simulink model "Projekt_FARE2_SS19_template_2015a"  (R2015a)
settings: Solver=ode4  SolverMode=SingleTasking  StartTime=0  StopTime=5  FixedStep=0.001  MaxStep=0.001  MinStep=1e-6  RelTol=1e-3  AbsTol=1e-3
PostLoadFcn:
  | %plot(Pos_x(:,2),Pos_y(:,2));
  | %xlabel('x(m)');
  | %ylabel('y(m)');
StopFcn:
  | %plot(Pos_x(:,2),Pos_y(:,2));
  | %xlabel('x(m)');
  | %ylabel('y(m)');
values from neighbouring files (symbols this model uses):
  delta_condi = 2    [init.m]
  K = place(A,B1,P)    [init.m]
  K10 = place(A10,B1,P)    [init.m]
  k3_condi = 1    [init.m]
  steig = 0.03    [init.m]
  v_condi = 0    [init.m]
  vorsteur_condi = 0    [init.m]
undefined symbols (not defined in the file or in its folder): in, sigbuilder_block
libraries: simulink x1
settings Model: Creator=vivgove  LastModifiedBy=eason
settings SolverCC: InitialStep=0.001  MaxOrder=3  AutoInsertRateTranBlk=on  InsertRTBMode=Never (minimum delay)
settings DataIOCC: LimitDataPoints=off  SignalLoggingSaveFormat=ModelDataLogs  SaveOutput=off  SignalLogging=off  SaveTime=off  OutputOption=SpecifiedOutputTimes  OutputTimes=[time]
settings OptimizationCC: InlineParams=on  ExpressionDepthLimit=2147483647  EfficientMapNaN2IntZero=off
settings DebuggingCC: UnderspecifiedInitializationDetection=Classic  MergeDetectMultiDrivingBlocksExec=none  SolverPrmCheckMsg=warning  FcnCallInpInsideContextMsg=EnableAllAsWarning  StateNameClashWarn=warning
settings HardwareCC: TargetBitPerLong=64  TargetBitPerPointer=64  TargetLongLongMode=on  TargetIntDivRoundTo=Zero  TargetEndianess=LittleEndian  TargetWordSize=64  TargetHWDeviceType=MATLAB Host  ProdEqTarget=off
settings CodeAppCC: MaxIdLength=128
settings GRTTargetCC: GeneratePreprocessorConditionals=Use local settings  CombineOutputUpdateFcns=off  GRTInterface=on

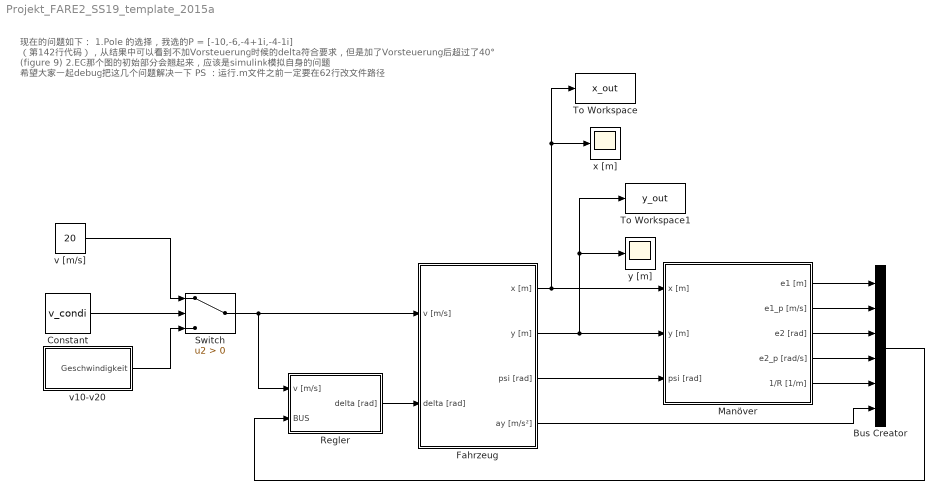
== system Projekt_FARE2_SS19_template_2015a ==
  note: 现在的问题如下：
      | 1.Pole 的选择，我选的P = [-10,-6,-4+1i,-4-1i] （第142行代码），从结果中可以看到不加Vorsteuerung时候的delta符合要求，但是加了Vorsteuerung后超过了40° (figure 9)
      | 2.EG那个图的初始部分会翘起来，应该是simulink模拟自身的问题
      |
      | 希望大家一起debug把这几个问题解决一下
      |
      | PS ：运行.m文件之前一定要在62行改文件路径
  Bus Creator : BusCreator  Inputs=6
  Constant : Constant  Value=v_condi
  Fahrzeug : Subsystem
  Manöver : Subsystem
  Regler : Subsystem
  Switch : Switch  Criteria=u2 > Threshold
  To Workspace : ToWorkspace  VariableName=x_out  SampleTime=-1
  To Workspace1 : ToWorkspace  VariableName=y_out  SampleTime=-1
  v [m/s] : Constant  Value=20
  v10-v20 : Subsystem  Tag=STV Subsys  LoadFcn=sigbuilder_block('load');  StartFcn=sigbuilder_block('start');  StopFcn=sigbuilder_block('stop');  ClipboardFcn=sigbuilder_block('clipboard');  mask(Sigbuilder block){}
      mask help: Simulink:masks:SigbuilderBlock_MD
      mask init:
      | if ~strcmp(get_param(bdroot(gcbh),'SimulationStatus'),'stopped') tuvar = sigbuilder_block('maskInit'); end
      settings: CopyFcn=sigbuilder_block('copy');  DeleteFcn=sigbuilder_block('delete');  ModelCloseFcn=sigbuilder_block('modelClose');  PreSaveFcn=sigbuilder_block('preSave');  PauseFcn=sigbuilder_block('pause');  ContinueFcn=sigbuilder_block('continue');  NameChangeFcn=sigbuilder_block('namechange');  OpenFcn=sigbuilder_block('open',[437.6 199.2 550.4 400 ]);  CloseFcn=sigbuilder_block('close');
      mask Display: plot(0, 0, 100, 100,[2, 2, 32, 32, 2], [68, 8, 8, 68, 68],[32, 2], [38, 38], [32, 19, 2],[53, 60, 44], [32, 17, 17, 2],[16, 16, 31, 31]);txt = getActiveGroup(gcbh);text(2, 100, txt,'verticalAlignment', 'top');
  x [m] : Scope
      settings: TimeRange=auto  MaxDataPoints=5000  SaveName=Pos_x  YMin=-9.34293  YMax=84.08636  SampleTime=-1  DataFormat=Array
  y [m] : Scope
      settings: TimeRange=auto  MaxDataPoints=5000  SaveName=Pos_y  YMin=-1.28728  YMax=1.75939  SampleTime=-1  DataFormat=Array
  wires:
  Manöver/1(e1 [m]) -> Bus Creator/1
  Manöver/2(e1_p [m/s]) -> Bus Creator/2
  Manöver/3(e2 [rad]) -> Bus Creator/3
  Manöver/4(e2_p [rad/s]) -> Bus Creator/4
  Manöver/5(1/R [1/m]) -> Bus Creator/5
  Bus Creator/1 -> Regler/2(BUS)
  Fahrzeug/1(x [m]) -> Manöver/1(x [m]), To Workspace/1, x [m]/1
  Fahrzeug/2(y [m]) -> Manöver/2(y [m]), y [m]/1, To Workspace1/1
  Regler/1(delta [rad]) -> Fahrzeug/2(delta [rad])
  Fahrzeug/3(psi [rad]) -> Manöver/3(psi [rad])
  Fahrzeug/4(ay [m/s²]) -> Bus Creator/6
  Switch/1 -> Fahrzeug/1(v [m/s]), Regler/1(v [m/s])
  Constant/1 -> Switch/2
  v [m/s]/1 -> Switch/1
  v10-v20/1(Geschwindigkeit) -> Switch/3

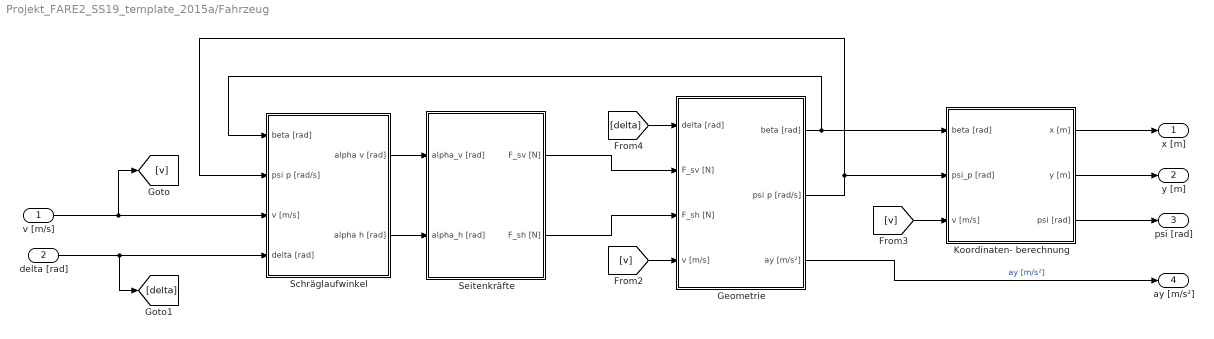
== system Projekt_FARE2_SS19_template_2015a/Fahrzeug ==
  v [m/s] : Inport
  delta [rad] : Inport  Port=2
  Geometrie : Subsystem
  Koordinaten- berechnung : Subsystem
  Schräglaufwinkel : Subsystem
  Seitenkräfte : Subsystem
  x [m] : Outport
  y [m] : Outport  Port=2
  psi [rad] : Outport  Port=3
  ay [m/s²] : Outport  Port=4
  wires:
  [v] -> Koordinaten- berechnung/3(v [m/s])
  delta [rad]/1 -> Schräglaufwinkel/4(delta [rad]), [delta]
  [v] -> Geometrie/4(v [m/s])
  [delta] -> Geometrie/1(delta [rad])
  v [m/s]/1 -> Schräglaufwinkel/3(v [m/s]), [v]
  Seitenkräfte/2(F_sh [N]) -> Geometrie/3(F_sh [N])
  Koordinaten- berechnung/3(psi [rad]) -> psi [rad]/1
  Koordinaten- berechnung/1(x [m]) -> x [m]/1
  Geometrie/2(psi p [rad/s]) -> Schräglaufwinkel/2(psi p [rad/s]), Koordinaten- berechnung/2(psi_p [rad])
  Schräglaufwinkel/2(alpha h [rad]) -> Seitenkräfte/2(alpha_h [rad])
  Koordinaten- berechnung/2(y [m]) -> y [m]/1
  Seitenkräfte/1(F_sv [N]) -> Geometrie/2(F_sv [N])
  Geometrie/1(beta [rad]) -> Koordinaten- berechnung/1(beta [rad]), Schräglaufwinkel/1(beta [rad])
  Schräglaufwinkel/1(alpha v [rad]) -> Seitenkräfte/1(alpha_v [rad])
  Geometrie/3(ay [m/s²]) -> ay [m/s²]/1  "ay [m/s²]"

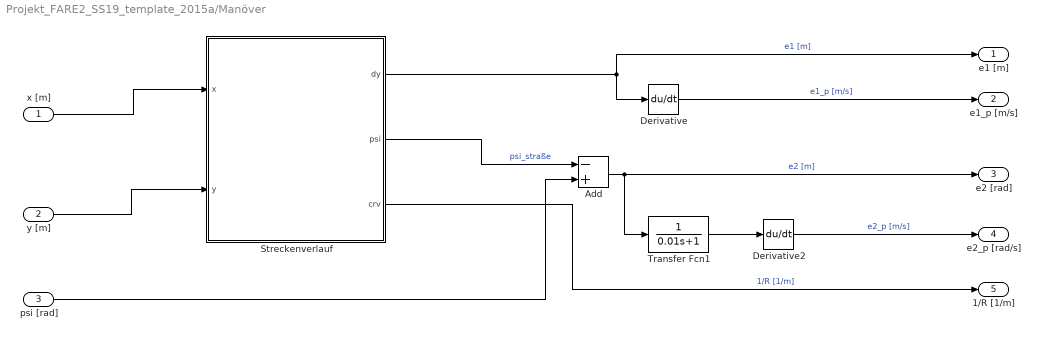
== system Projekt_FARE2_SS19_template_2015a/Manöver ==
  x [m] : Inport
  y [m] : Inport  Port=2
  psi [rad] : Inport  Port=3
  Add : Sum  Inputs=-+
  Derivative : Derivative
  Derivative2 : Derivative
  Streckenverlauf : MATLAB Function  TreatAsAtomicUnit=on
      settings: PermitHierarchicalResolution=ParametersOnly
  Transfer Fcn1 : TransferFcn  Denominator=[0.01 1]
  e1 [m] : Outport
  e1_p [m/s] : Outport  Port=2
  e2 [rad] : Outport  Port=3
  e2_p [rad/s] : Outport  Port=4
  1/R [1/m] : Outport  Port=5
  wires:
  Streckenverlauf/3(crv) -> 1/R [1/m]/1  "1/R [1/m]"
  Streckenverlauf/2(psi) -> Add/1  "psi_straße"
  Streckenverlauf/1(dy) -> e1 [m]/1, Derivative/1  "e1 [m]"
  psi [rad]/1 -> Add/2
  Add/1 -> e2 [rad]/1, Transfer Fcn1/1  "e2 [m]"
  Derivative2/1 -> e2_p [rad/s]/1  "e2_p [m/s]"
  Transfer Fcn1/1 -> Derivative2/1
  y [m]/1 -> Streckenverlauf/2(y)
  Derivative/1 -> e1_p [m/s]/1  "e1_p [m/s]"
  x [m]/1 -> Streckenverlauf/1(x)

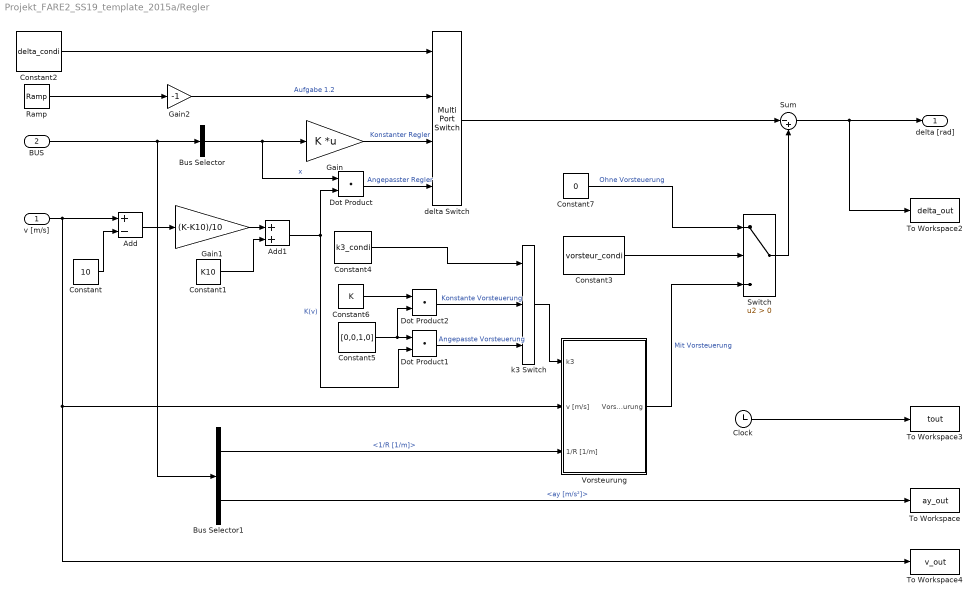
== system Projekt_FARE2_SS19_template_2015a/Regler ==
  v [m/s] : Inport
  BUS : Inport  Port=2
  Add : Sum  Inputs=+-
  Add1 : Sum  Inputs=2
  Bus Selector : BusSelector  OutputSignals=e1 [m],e1_p [m/s],e2 [m],e2_p [m/s]  OutputAsBus=on
  Bus Selector1 : BusSelector  OutputSignals=1/R [1/m],ay [m/s²]
  Clock : Clock
  Constant : Constant  Value=10
  Constant1 : Constant  Value=K10
  Constant2 : Constant  Value=delta_condi
  Constant3 : Constant  Value=vorsteur_condi
  Constant4 : Constant  Value=k3_condi
  Constant5 : Constant  Value=[0,0,1,0]
  Constant6 : Constant  Value=K
  Constant7 : Constant  Value=0
  Dot Product : DotProduct  InputSameDT=on  OutDataTypeStr=Inherit: Inherit via internal rule
  Dot Product1 : DotProduct  InputSameDT=on  OutDataTypeStr=Inherit: Inherit via internal rule
  Dot Product2 : DotProduct  InputSameDT=on  OutDataTypeStr=Inherit: Inherit via internal rule
  Gain : Gain  Gain=K  Multiplication=Matrix(K*u) (u vector)
  Gain1 : Gain  Gain=(K-K10)/10
  Gain2 : Gain  Gain=-1
  Ramp : simulink/Sources/Ramp  slope=steig  start=0  X0=0
  Sum : Sum  Inputs=|-+
  Switch : Switch  Criteria=u2 > Threshold
  To Workspace : ToWorkspace  VariableName=ay_out  SampleTime=-1
  To Workspace2 : ToWorkspace  VariableName=delta_out  SampleTime=-1
  To Workspace3 : ToWorkspace  VariableName=tout  SampleTime=-1
  To Workspace4 : ToWorkspace  VariableName=v_out  SampleTime=-1
  Vorsteurung : Subsystem
  delta Switch : MultiPortSwitch
  k3 Switch : MultiPortSwitch  Inputs=2
  delta [rad] : Outport
  wires:
  BUS/1 -> Bus Selector/1, Bus Selector1/1
  Bus Selector/1 -> Gain/1, Dot Product/1  "x"
  Sum/1 -> To Workspace2/1, delta [rad]/1
  Constant/1 -> Add/2
  Add/1 -> Gain1/1
  Gain1/1 -> Add1/1
  Constant1/1 -> Add1/2
  Gain/1 -> delta Switch/3  "Konstanter Regler"
  Ramp/1 -> Gain2/1
  Dot Product/1 -> delta Switch/4  "Angepasster Regler"
  Add1/1 -> Dot Product1/2, Dot Product/2  "K(v)"
  delta Switch/1 -> Sum/1
  Constant2/1 -> delta Switch/1
  Bus Selector1/1 -> Vorsteurung/3(1/R [1/m])  "<1/R [1/m]>"
  Bus Selector1/2 -> To Workspace/1  "<ay [m/s²]>"
  Constant5/1 -> Dot Product2/2, Dot Product1/1
  Clock/1 -> To Workspace3/1
  v [m/s]/1 -> To Workspace4/1, Vorsteurung/2(v [m/s]), Add/1
  Gain2/1 -> delta Switch/2  "Aufgabe 1.2"
  Constant6/1 -> Dot Product2/1
  k3 Switch/1 -> Vorsteurung/1(k3)
  Dot Product2/1 -> k3 Switch/2  "Konstante Vorsteuerung"
  Dot Product1/1 -> k3 Switch/3  "Angepasste Vorsteuerung"
  Constant4/1 -> k3 Switch/1
  Constant3/1 -> Switch/2
  Constant7/1 -> Switch/1  "Ohne Vorsteuerung"
  Vorsteurung/1(Vorsteurung) -> Switch/3  "Mit Vorsteuerung"
  Switch/1 -> Sum/2

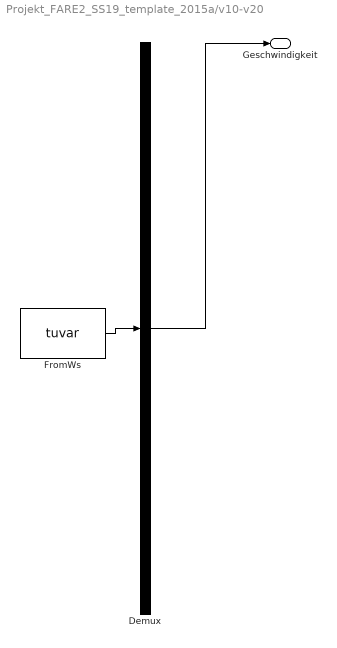
== system Projekt_FARE2_SS19_template_2015a/v10-v20 ==
  Demux : Demux  Tag=STV Demux  Outputs=1
  FromWs : FromWorkspace  Tag=STV FromWs  VariableName=tuvar  SampleTime=0
      SigBuilderData=|
      | common.afterFinalStr = 'Extrapolate'
      | common.sampleTime = 0
      | dataSet.timeRange = [0 5]
      | dataSet.name = 'Group 1'
      | sbobj.Groups.Name = 'Group 1'
      | sbobj.Groups.Signals.Name = 'Geschwindigkeit'
      | sbobj.Groups.Signals.XData = [0 2.5 5]
      | sbobj.Groups.Signals.YData = [10 13.35 20]
      | sbobj.Groups.TimeRange = [0 5]
  Geschwindigkeit : Outport  Tag=STV Outport
  wires:
  Demux/1 -> Geschwindigkeit/1
  FromWs/1 -> Demux/1

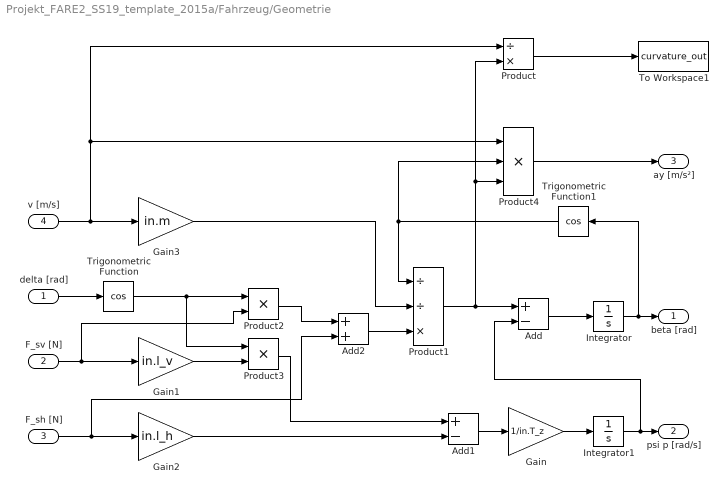
== system Projekt_FARE2_SS19_template_2015a/Fahrzeug/Geometrie ==
  delta [rad] : Inport
  F_sv [N] : Inport  Port=2
  F_sh [N] : Inport  Port=3
  v [m/s] : Inport  Port=4
  Add : Sum  Inputs=+-
  Add1 : Sum  Inputs=+-
  Add2 : Sum  Inputs=2
  Gain : Gain  Gain=1/in.T_z
  Gain1 : Gain  Gain=in.l_v
  Gain2 : Gain  Gain=in.l_h
  Gain3 : Gain  Gain=in.m
  Integrator : Integrator
  Integrator1 : Integrator
  Product : Product  Inputs=/*
  Product1 : Product  Inputs=//*
  Product2 : Product
  Product3 : Product
  Product4 : Product  Inputs=3
  To Workspace1 : ToWorkspace  VariableName=curvature_out  SampleTime=-1
  Trigonometric Function : Trigonometry  Operator=cos
  Trigonometric Function1 : Trigonometry  Operator=cos
  beta [rad] : Outport
  psi p [rad/s] : Outport  Port=2
  ay [m/s²] : Outport  Port=3
  wires:
  v [m/s]/1 -> Product4/1, Product/1, Gain3/1
  delta [rad]/1 -> Trigonometric Function/1
  F_sh [N]/1 -> Add2/2, Gain2/1
  Integrator/1 -> beta [rad]/1, Trigonometric Function1/1
  Add/1 -> Integrator/1
  Integrator1/1 -> Add/2, psi p [rad/s]/1
  Product1/1 -> Product/2, Product4/3, Add/1
  Gain/1 -> Integrator1/1
  Add1/1 -> Gain/1
  F_sv [N]/1 -> Product2/2, Gain1/1
  Gain1/1 -> Product3/2
  Trigonometric Function/1 -> Product3/1, Product2/1
  Product3/1 -> Add1/1
  Gain2/1 -> Add1/2
  Gain3/1 -> Product1/2
  Trigonometric Function1/1 -> Product4/2, Product1/1
  Product2/1 -> Add2/1
  Add2/1 -> Product1/3
  Product4/1 -> ay [m/s²]/1
  Product/1 -> To Workspace1/1

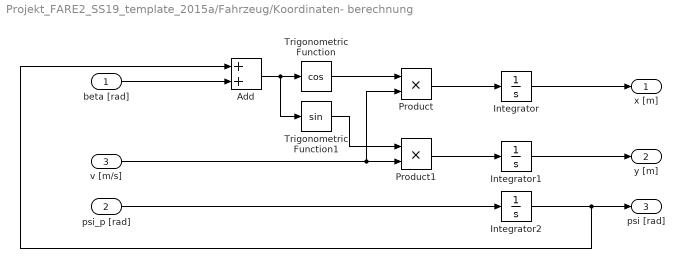
== system Projekt_FARE2_SS19_template_2015a/Fahrzeug/Koordinaten- berechnung ==
  beta [rad] : Inport
  psi_p [rad] : Inport  Port=2
  v [m/s] : Inport  Port=3
  Add : Sum
  Integrator : Integrator
  Integrator1 : Integrator
  Integrator2 : Integrator
  Product : Product
  Product1 : Product
  Trigonometric Function : Trigonometry  Operator=cos
  Trigonometric Function1 : Trigonometry
  x [m] : Outport
  y [m] : Outport  Port=2
  psi [rad] : Outport  Port=3
  wires:
  psi_p [rad]/1 -> Integrator2/1
  beta [rad]/1 -> Add/2
  Integrator1/1 -> y [m]/1
  Integrator2/1 -> Add/1, psi [rad]/1
  Add/1 -> Trigonometric Function1/1, Trigonometric Function/1
  Product/1 -> Integrator/1
  Trigonometric Function/1 -> Product/1
  Product1/1 -> Integrator1/1
  v [m/s]/1 -> Product/2, Product1/2
  Trigonometric Function1/1 -> Product1/1
  Integrator/1 -> x [m]/1

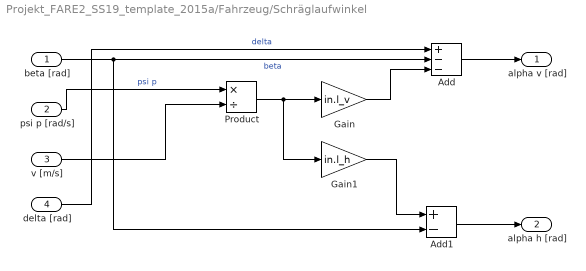
== system Projekt_FARE2_SS19_template_2015a/Fahrzeug/Schräglaufwinkel ==
  beta [rad] : Inport
  psi p [rad/s] : Inport  Port=2
  v [m/s] : Inport  Port=3
  delta [rad] : Inport  Port=4
  Add : Sum  Inputs=+--
  Add1 : Sum  Inputs=+-
  Gain : Gain  Gain=in.l_v
  Gain1 : Gain  Gain=in.l_h
  Product : Product  Inputs=*/
  alpha v [rad] : Outport
  alpha h [rad] : Outport  Port=2
  wires:
  beta [rad]/1 -> Add1/2, Add/2  "beta"
  delta [rad]/1 -> Add/1  "delta"
  psi p [rad/s]/1 -> Product/1  "psi p"
  Add/1 -> alpha v [rad]/1
  Add1/1 -> alpha h [rad]/1
  v [m/s]/1 -> Product/2
  Product/1 -> Gain1/1, Gain/1
  Gain/1 -> Add/3
  Gain1/1 -> Add1/1

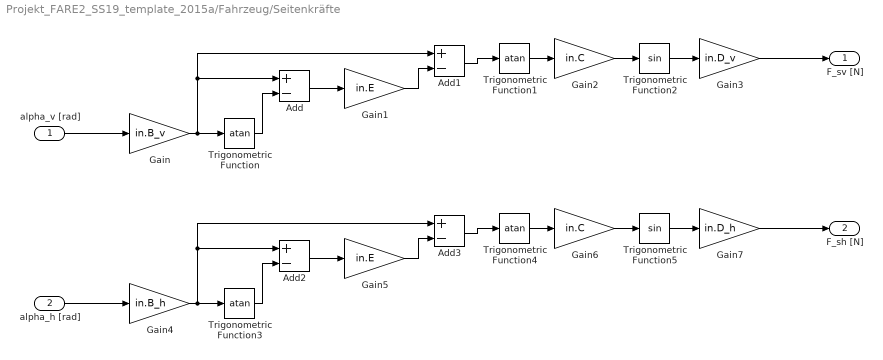
== system Projekt_FARE2_SS19_template_2015a/Fahrzeug/Seitenkräfte ==
  alpha_v [rad] : Inport
  alpha_h [rad] : Inport  Port=2
  Add{,1..3} (4 alike) : Sum  Inputs=+-
  Gain : Gain  Gain=in.B_v
  Gain1 : Gain  Gain=in.E
  Gain2 : Gain  Gain=in.C
  Gain3 : Gain  Gain=in.D_v
  Gain4 : Gain  Gain=in.B_h
  Gain5 : Gain  Gain=in.E
  Gain6 : Gain  Gain=in.C
  Gain7 : Gain  Gain=in.D_h
  Trigonometric Function{,1,3..4} (4 alike) : Trigonometry  Operator=atan
  Trigonometric Function2 : Trigonometry
  Trigonometric Function5 : Trigonometry
  F_sv [N] : Outport
  F_sh [N] : Outport  Port=2
  wires:
  alpha_v [rad]/1 -> Gain/1
  Gain3/1 -> F_sv [N]/1
  Gain/1 -> Trigonometric Function/1, Add1/1, Add/1
  Trigonometric Function/1 -> Add/2
  Add/1 -> Gain1/1
  Gain1/1 -> Add1/2
  Add1/1 -> Trigonometric Function1/1
  Trigonometric Function1/1 -> Gain2/1
  Gain2/1 -> Trigonometric Function2/1
  Trigonometric Function2/1 -> Gain3/1
  alpha_h [rad]/1 -> Gain4/1
  Gain4/1 -> Trigonometric Function3/1, Add3/1, Add2/1
  Trigonometric Function3/1 -> Add2/2
  Add2/1 -> Gain5/1
  Gain5/1 -> Add3/2
  Add3/1 -> Trigonometric Function4/1
  Trigonometric Function4/1 -> Gain6/1
  Gain6/1 -> Trigonometric Function5/1
  Trigonometric Function5/1 -> Gain7/1
  Gain7/1 -> F_sh [N]/1

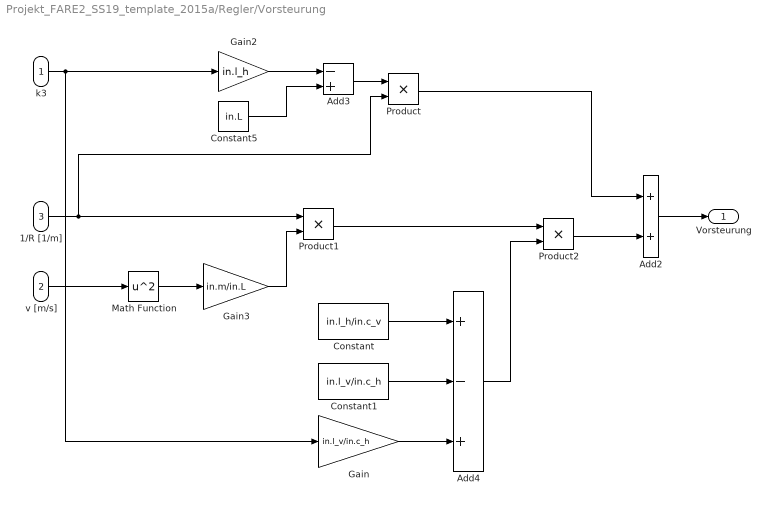
== system Projekt_FARE2_SS19_template_2015a/Regler/Vorsteurung ==
  k3 : Inport
  v [m/s] : Inport  Port=2
  1/R [1/m] : Inport  Port=3
  Add2 : Sum
  Add3 : Sum  Inputs=-+
  Add4 : Sum  Inputs=+-+
  Constant : Constant  Value=in.l_h/in.c_v
  Constant1 : Constant  Value=in.l_v/in.c_h
  Constant5 : Constant  Value=in.L
  Gain : Gain  Gain=in.l_v/in.c_h
  Gain2 : Gain  Gain=in.l_h
  Gain3 : Gain  Gain=in.m/in.L
  Math Function : Math  Operator=square  SaturateOnIntegerOverflow=on
  Product : Product
  Product1 : Product
  Product2 : Product
  Vorsteurung : Outport
  wires:
  k3/1 -> Gain/1, Gain2/1
  1/R [1/m]/1 -> Product1/1, Product/2
  Product1/1 -> Product2/1
  Add2/1 -> Vorsteurung/1
  Add4/1 -> Product2/2
  Constant5/1 -> Add3/2
  Product/1 -> Add2/1
  Gain2/1 -> Add3/1
  Add3/1 -> Product/1
  Constant1/1 -> Add4/2
  Gain/1 -> Add4/3
  Constant/1 -> Add4/1
  Product2/1 -> Add2/2
  Math Function/1 -> Gain3/1
  Gain3/1 -> Product1/2
  v [m/s]/1 -> Math Function/1

== matlab function Projekt_FARE2_SS19_template_2015a/Manöver/Streckenverlauf ==
  data: x input; data parameter; dy output; y input; psi output; crv output
function  [dy,psi,crv] = Berechnung_Streckendaten(x,data,y)
%#codegen

puv=crg_eval_xy2uv_adaptiert(data, [x y]);
psi=crg_eval_u2phi(data, puv(1));
crv=crg_eval_u2crv(data, puv(1));
dy=puv(2);
